simulink model "mrefrobotarm_modified_previous_y_previous_u_previous_ref_Thao"  (R2018b)
settings: Solver=FixedStepAuto  StartTime=0.0  StopTime=10  RelTol=1e-3  AbsTol=1e-6
undefined symbols (not defined in the file or in its folder): sfunxy2
libraries: neural x668, simulink x1
(part 14 of 21)

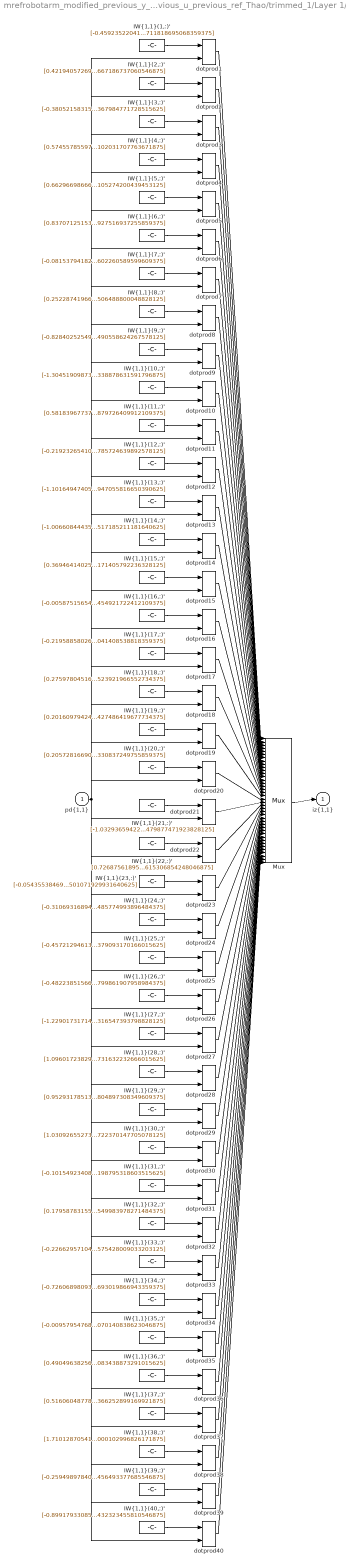
== system mrefrobotarm_modified_previous_y_previous_u_previous_ref_Thao/trimmed_1/Layer 1/IW{1,1} ==
  "pd{1,1}" : Inport  PortDimensions=10
      mask Display: e = 0.06;c1 = [120 230 180]/255;c2 = ([120 230 180]+0)/(256+128);c3 = ([120 230 180]+128)/(256+128);patch([0 1 1 0],[0 0 1 1],c1);patch([0 1 1 1-e 1-e 0+e],[0 0 1 1-e 0+e 0+e],c2);patch([0 0 1 1-e 0+e 0+e],[0 1 1 1-e 1-e 0+e],c3);plot([0 1 1 0 0],[0 0 1 1 0]);
  "IW{1,1}(1,:)'" : Constant  Value=[-0.459235220416795819620148222384159453213214874267578125;-0.29349824568717675088436180885764770209789276123046875;1.04961602685572064075358866830356419086456298828125;0.7919521211983930886191274112206883728504180908203125;-1.1784595378789595176982629709527827799320220947265625;1.1211787526460994524057923626969568431377410888671875;-0.490550798188298220470215937893954105675220489501953125;0.0281424900047358324262081197275620070286095142364501953125;0.443160657725568507547819763203733600676059722900390625;-0.1531042527124218677325728776850155554711818695068359375]
      mask Display: e = 0.06;c1 = [120 150 230]/255;c2 = ([120 150 230]+0)/383;c3 = ([120 150 230]+128)/383;patch([0 1 1 0],[0 0 1 1],c1);patch([0 1 1 1-e 1-e 0+e],[0 0 1 1-e 0+e 0+e],c2);patch([0 0 1 1-e 0+e 0+e],[0 1 1 1-e 1-e 0+e],c3);plot([0 1 1 0 0],[0 0 1 1 0]);disp('Weights');
  "IW{1,1}(10,:)'" : Constant  Value=[-1.304519098736843130126317191752605140209197998046875;-0.306877759776605751884659412098699249327182769775390625;0.5237566266513227208889702524174936115741729736328125;0.10945152834388600926462942197758820839226245880126953125;0.48910555309599768047945644866558723151683807373046875;-1.0719933374810057813419916783459484577178955078125;-0.15974131494668253328228502141428180038928985595703125;0.804989926550838230667750394786708056926727294921875;-0.046877573285782979384261892619178979657590389251708984375;-0.060441319600902036757172908210122841410338878631591796875]
      mask Display: e = 0.06;c1 = [120 150 230]/255;c2 = ([120 150 230]+0)/383;c3 = ([120 150 230]+128)/383;patch([0 1 1 0],[0 0 1 1],c1);patch([0 1 1 1-e 1-e 0+e],[0 0 1 1-e 0+e 0+e],c2);patch([0 0 1 1-e 0+e 0+e],[0 1 1 1-e 1-e 0+e],c3);plot([0 1 1 0 0],[0 0 1 1 0]);disp('Weights');
  "IW{1,1}(11,:)'" : Constant  Value=[0.5818396773725129644816433938103727996349334716796875;-0.0152744671885454534610015997486698324792087078094482421875;-1.3902737988604008112503152005956508219242095947265625;-0.090341627385831457797138455134700052440166473388671875;-0.08192938236897930048829863380888127721846103668212890625;-1.1836377842268201998621179882320575416088104248046875;-0.94837696822625761061686944231041707098484039306640625;0.67302924934781593879762340293382294476032257080078125;0.279503475348413743528652730674366466701030731201171875;-0.7270775313874044964990162043250165879726409912109375]
      mask Display: e = 0.06;c1 = [120 150 230]/255;c2 = ([120 150 230]+0)/383;c3 = ([120 150 230]+128)/383;patch([0 1 1 0],[0 0 1 1],c1);patch([0 1 1 1-e 1-e 0+e],[0 0 1 1-e 0+e 0+e],c2);patch([0 0 1 1-e 0+e 0+e],[0 1 1 1-e 1-e 0+e],c3);plot([0 1 1 0 0],[0 0 1 1 0]);disp('Weights');
  "IW{1,1}(12,:)'" : Constant  Value=[-0.2192326541079176183135501787546672858297824859619140625;0.034961204740979488769792027369476272724568843841552734375;-0.78480877090928391481838843901641666889190673828125;-0.68497188483738924436039496868033893406391143798828125;0.9496056043739018459604039890109561383724212646484375;0.59138070807167919529234723086119629442691802978515625;0.02938148514822198908991168764259782619774341583251953125;0.47042016217384075016383349066018126904964447021484375;0.0528506255461557439279118852937244810163974761962890625;0.8492892171110704158110138450865633785724639892578125]
      mask Display: e = 0.06;c1 = [120 150 230]/255;c2 = ([120 150 230]+0)/383;c3 = ([120 150 230]+128)/383;patch([0 1 1 0],[0 0 1 1],c1);patch([0 1 1 1-e 1-e 0+e],[0 0 1 1-e 0+e 0+e],c2);patch([0 0 1 1-e 0+e 0+e],[0 1 1 1-e 1-e 0+e],c3);plot([0 1 1 0 0],[0 0 1 1 0]);disp('Weights');
  "IW{1,1}(13,:)'" : Constant  Value=[-1.1016494740575859534459368660463951528072357177734375;-0.58886092713398652254142007222981192171573638916015625;-0.7307837342220271370507589381304569542407989501953125;0.7557155236138466403161828566226176917552947998046875;-0.34920491976783851750809617442428134381771087646484375;-0.87052916654144818497940150336944498121738433837890625;-0.1667532157244010215801921503953053615987300872802734375;-0.054286569446526149185228149463000590912997722625732421875;0.241223838878424856613236215707729570567607879638671875;0.700996124572663692475771313183940947055816650390625]
      mask Display: e = 0.06;c1 = [120 150 230]/255;c2 = ([120 150 230]+0)/383;c3 = ([120 150 230]+128)/383;patch([0 1 1 0],[0 0 1 1],c1);patch([0 1 1 1-e 1-e 0+e],[0 0 1 1-e 0+e 0+e],c2);patch([0 0 1 1-e 0+e 0+e],[0 1 1 1-e 1-e 0+e],c3);plot([0 1 1 0 0],[0 0 1 1 0]);disp('Weights');
  "IW{1,1}(14,:)'" : Constant  Value=[-1.006608444357844245331534693832509219646453857421875;-0.35711572844715055996545061134384013712406158447265625;0.32909480035113836127180775292799808084964752197265625;-0.55110276961780180204897305884514935314655303955078125;1.154802213522362563935530488379299640655517578125;0.397605348225490207170196299557574093341827392578125;-0.71574591313160329519860169966705143451690673828125;0.48159191024112935064493967729504220187664031982421875;-0.78679680756141412434345738802221603691577911376953125;-0.441768530810494441940505794264026917517185211181640625]
      mask Display: e = 0.06;c1 = [120 150 230]/255;c2 = ([120 150 230]+0)/383;c3 = ([120 150 230]+128)/383;patch([0 1 1 0],[0 0 1 1],c1);patch([0 1 1 1-e 1-e 0+e],[0 0 1 1-e 0+e 0+e],c2);patch([0 0 1 1-e 0+e 0+e],[0 1 1 1-e 1-e 0+e],c3);plot([0 1 1 0 0],[0 0 1 1 0]);disp('Weights');
  "IW{1,1}(15,:)'" : Constant  Value=[0.369464140250917616459247483362560160458087921142578125;-0.937888588280831658750003043678589165210723876953125;1.0867534228885114000462408512248657643795013427734375;-0.52592004088093335933962180206435732543468475341796875;0.112207093713337424656373286779853515326976776123046875;0.465684224635162069549920715871849097311496734619140625;-0.431210336591754950230637177810422144830226898193359375;-0.303101408244178305295690734055824577808380126953125;-0.69731111958409119910839990552631206810474395751953125;0.08481772702666075247623922450657119043171405792236328125]
      mask Display: e = 0.06;c1 = [120 150 230]/255;c2 = ([120 150 230]+0)/383;c3 = ([120 150 230]+128)/383;patch([0 1 1 0],[0 0 1 1],c1);patch([0 1 1 1-e 1-e 0+e],[0 0 1 1-e 0+e 0+e],c2);patch([0 0 1 1-e 0+e 0+e],[0 1 1 1-e 1-e 0+e],c3);plot([0 1 1 0 0],[0 0 1 1 0]);disp('Weights');
  "IW{1,1}(16,:)'" : Constant  Value=[-0.005875156547677277962815622913694824092090129852294921875;-0.77071460027049354390982216500560753047466278076171875;-1.142444277782478589955417191958986222743988037109375;0.00057501630162004428725719407111682812683284282684326171875;1.1843998886999156372468178233248181641101837158203125;-0.564351201026638715774197407881729304790496826171875;-0.6111872289272748393074152772896923124790191650390625;-0.6547030283798418448526490465155802667140960693359375;-1.1908742302352506303719792413176037371158599853515625;-0.0548431276366504183439332109628594480454921722412109375]
      mask Display: e = 0.06;c1 = [120 150 230]/255;c2 = ([120 150 230]+0)/383;c3 = ([120 150 230]+128)/383;patch([0 1 1 0],[0 0 1 1],c1);patch([0 1 1 1-e 1-e 0+e],[0 0 1 1-e 0+e 0+e],c2);patch([0 0 1 1-e 0+e 0+e],[0 1 1 1-e 1-e 0+e],c3);plot([0 1 1 0 0],[0 0 1 1 0]);disp('Weights');
  "IW{1,1}(17,:)'" : Constant  Value=[-0.2195885802646860562870045896488591097295284271240234375;-0.3575806967372410216654543546610511839389801025390625;0.97143694571848226981813922975561581552028656005859375;-0.8289197498612617120983259155764244496822357177734375;-0.5746253167151700314008166969870217144489288330078125;-0.0506852139293310910428402848992845974862575531005859375;-0.2294990560698609016743176880481769330799579620361328125;0.416849708577010702459375579564948566257953643798828125;-0.87616338373132840455781433774973265826702117919921875;0.08519930707200072672602431111954501830041408538818359375]
      mask Display: e = 0.06;c1 = [120 150 230]/255;c2 = ([120 150 230]+0)/383;c3 = ([120 150 230]+128)/383;patch([0 1 1 0],[0 0 1 1],c1);patch([0 1 1 1-e 1-e 0+e],[0 0 1 1-e 0+e 0+e],c2);patch([0 0 1 1-e 0+e 0+e],[0 1 1 1-e 1-e 0+e],c3);plot([0 1 1 0 0],[0 0 1 1 0]);disp('Weights');
  "IW{1,1}(18,:)'" : Constant  Value=[0.275978045164061158711632515405653975903987884521484375;-0.201844925448067258333395557201583869755268096923828125;0.369878378264276774789465207504690624773502349853515625;0.413333003679872412750029297967557795345783233642578125;0.506360871776887488948659665766172111034393310546875;-0.93265275816585446744255705198156647384166717529296875;-0.0965695424353806008976874863947159610688686370849609375;0.36861066338864378888473538609105162322521209716796875;-0.734700546032511336846937410882674157619476318359375;-0.99055277611612291277509712017490528523921966552734375]
      mask Display: e = 0.06;c1 = [120 150 230]/255;c2 = ([120 150 230]+0)/383;c3 = ([120 150 230]+128)/383;patch([0 1 1 0],[0 0 1 1],c1);patch([0 1 1 1-e 1-e 0+e],[0 0 1 1-e 0+e 0+e],c2);patch([0 0 1 1-e 0+e 0+e],[0 1 1 1-e 1-e 0+e],c3);plot([0 1 1 0 0],[0 0 1 1 0]);disp('Weights');
  "IW{1,1}(19,:)'" : Constant  Value=[0.2016097942440719104073565404178225435316562652587890625;-0.292006737817900929865544412677991203963756561279296875;1.0762677103940505585200071436702273786067962646484375;-0.437529738725115524555775436965632252395153045654296875;1.4057628148362562026107980273081921041011810302734375;-1.0115085483930297272081588744185864925384521484375;1.4608491956607905226661614506156183779239654541015625;-0.0263676635064111104800321783159233746118843555450439453125;-0.560893447360877761553865639143623411655426025390625;0.01126831078487092706319483426113947643898427486419677734375]
      mask Display: e = 0.06;c1 = [120 150 230]/255;c2 = ([120 150 230]+0)/383;c3 = ([120 150 230]+128)/383;patch([0 1 1 0],[0 0 1 1],c1);patch([0 1 1 1-e 1-e 0+e],[0 0 1 1-e 0+e 0+e],c2);patch([0 0 1 1-e 0+e 0+e],[0 1 1 1-e 1-e 0+e],c3);plot([0 1 1 0 0],[0 0 1 1 0]);disp('Weights');
  "IW{1,1}(2,:)'" : Constant  Value=[0.421940572696684224052177114572259597480297088623046875;1.1394047830481301986083053634501993656158447265625;-0.9276428928608384527620955850579775869846343994140625;-0.319621581377210917107589693841873668134212493896484375;0.599161290037102833849758098949678242206573486328125;0.3502538826006265093582214831258170306682586669921875;0.76486814909031386466864432804868556559085845947265625;-0.39442526404542543883025018658372573554515838623046875;0.727514701167386146352100695366971194744110107421875;-0.276969707672654219532404340498032979667186737060546875]
      mask Display: e = 0.06;c1 = [120 150 230]/255;c2 = ([120 150 230]+0)/383;c3 = ([120 150 230]+128)/383;patch([0 1 1 0],[0 0 1 1],c1);patch([0 1 1 1-e 1-e 0+e],[0 0 1 1-e 0+e 0+e],c2);patch([0 0 1 1-e 0+e 0+e],[0 1 1 1-e 1-e 0+e],c3);plot([0 1 1 0 0],[0 0 1 1 0]);disp('Weights');
  "IW{1,1}(20,:)'" : Constant  Value=[0.205728166907649556716108918408281169831752777099609375;0.98978059918219962742824691304122097790241241455078125;0.670105035888260314180797649896703660488128662109375;-0.0727233259149407673671561269657104276120662689208984375;1.153059473829215253459778978140093386173248291015625;0.491497972255601933699864503068965859711170196533203125;-0.69500217773896599826599640437052585184574127197265625;0.85994847944253038907191921680350787937641143798828125;-0.835551186472724527476430012029595673084259033203125;-0.74790216150634802882990470607182942330837249755859375]
      mask Display: e = 0.06;c1 = [120 150 230]/255;c2 = ([120 150 230]+0)/383;c3 = ([120 150 230]+128)/383;patch([0 1 1 0],[0 0 1 1],c1);patch([0 1 1 1-e 1-e 0+e],[0 0 1 1-e 0+e 0+e],c2);patch([0 0 1 1-e 0+e 0+e],[0 1 1 1-e 1-e 0+e],c3);plot([0 1 1 0 0],[0 0 1 1 0]);disp('Weights');
  "IW{1,1}(21,:)'" : Constant  Value=[-1.0329365942279211676435579647659324109554290771484375;0.42458628807360121459879565009032376110553741455078125;0.04618443901148210073426270128038595430552959442138671875;0.9065560967748407250610398477874696254730224609375;0.26648361510755302905550934156053699553012847900390625;0.0884291687942552473433721615947433747351169586181640625;0.61770434825117381816284023443586193025112152099609375;0.4629829983966817774643232041853480041027069091796875;-1.0141119299122414165736927316174842417240142822265625;0.15100917945186254076617160535533912479877471923828125]
      mask Display: e = 0.06;c1 = [120 150 230]/255;c2 = ([120 150 230]+0)/383;c3 = ([120 150 230]+128)/383;patch([0 1 1 0],[0 0 1 1],c1);patch([0 1 1 1-e 1-e 0+e],[0 0 1 1-e 0+e 0+e],c2);patch([0 0 1 1-e 0+e 0+e],[0 1 1 1-e 1-e 0+e],c3);plot([0 1 1 0 0],[0 0 1 1 0]);disp('Weights');
  "IW{1,1}(22,:)'" : Constant  Value=[0.7268756189553073898679258491029031574726104736328125;-0.467689105554118522700690618876251392066478729248046875;1.109281880772417405722762850928120315074920654296875;0.27315022414110179393986754803336225450038909912109375;0.43094504121100218885231925014522857964038848876953125;-0.163097227005093603491303611008333973586559295654296875;0.86284083669027011875840571519802324473857879638671875;0.44549143038833693974964944573002867400646209716796875;0.299238776986608112640197987275314517319202423095703125;-1.12148762799542378587602797779254615306854248046875]
      mask Display: e = 0.06;c1 = [120 150 230]/255;c2 = ([120 150 230]+0)/383;c3 = ([120 150 230]+128)/383;patch([0 1 1 0],[0 0 1 1],c1);patch([0 1 1 1-e 1-e 0+e],[0 0 1 1-e 0+e 0+e],c2);patch([0 0 1 1-e 0+e 0+e],[0 1 1 1-e 1-e 0+e],c3);plot([0 1 1 0 0],[0 0 1 1 0]);disp('Weights');
  "IW{1,1}(23,:)'" : Constant  Value=[-0.0543553846922637806660105752598610706627368927001953125;0.0894024321997811954876311801854171790182590484619140625;-0.73268180455055631483674005721695721149444580078125;-0.87990063776815652385465682527865283191204071044921875;-0.1341766531305843279664458123079384677112102508544921875;0.617144986876134726827558552031405270099639892578125;-0.64440139361752535318572654432500712573528289794921875;-0.5619417681658263052923985014786012470722198486328125;-1.0054577554698818087075551375164650380611419677734375;-0.64369874313411801214357410572119988501071929931640625]
      mask Display: e = 0.06;c1 = [120 150 230]/255;c2 = ([120 150 230]+0)/383;c3 = ([120 150 230]+128)/383;patch([0 1 1 0],[0 0 1 1],c1);patch([0 1 1 1-e 1-e 0+e],[0 0 1 1-e 0+e 0+e],c2);patch([0 0 1 1-e 0+e 0+e],[0 1 1 1-e 1-e 0+e],c3);plot([0 1 1 0 0],[0 0 1 1 0]);disp('Weights');
  "IW{1,1}(24,:)'" : Constant  Value=[-0.31069316894714871235549935590825043618679046630859375;-0.5814084330997444372002291856915690004825592041015625;-0.822688715191450814501195054617710411548614501953125;-0.1990172295149660597335383727113367058336734771728515625;-0.253642741079357747491229702063719742000102996826171875;1.2263993908007790878400555811822414398193359375;-1.0833193209512239629788155070855282247066497802734375;-0.7328344121728693760786654820549301803112030029296875;-0.466145811881534422038697584866895340383052825927734375;0.67576516762366212187629344043671153485774993896484375]
      mask Display: e = 0.06;c1 = [120 150 230]/255;c2 = ([120 150 230]+0)/383;c3 = ([120 150 230]+128)/383;patch([0 1 1 0],[0 0 1 1],c1);patch([0 1 1 1-e 1-e 0+e],[0 0 1 1-e 0+e 0+e],c2);patch([0 0 1 1-e 0+e 0+e],[0 1 1 1-e 1-e 0+e],c3);plot([0 1 1 0 0],[0 0 1 1 0]);disp('Weights');
  "IW{1,1}(25,:)'" : Constant  Value=[-0.457212946136130060637015048996545374393463134765625;-0.7632016106977881353401471642428077757358551025390625;0.248761073438853286265981523683876730501651763916015625;-0.82845030997187818488924904158920980989933013916015625;0.505824858023265822026814930723048746585845947265625;-0.07525956372700999541525135327901807613670825958251953125;-0.43507647282099137786559595042490400373935699462890625;0.1433382425757481204442456146352924406528472900390625;-1.012707980842789456943364712060429155826568603515625;1.0154921878932070544721000260324217379093170166015625]
      mask Display: e = 0.06;c1 = [120 150 230]/255;c2 = ([120 150 230]+0)/383;c3 = ([120 150 230]+128)/383;patch([0 1 1 0],[0 0 1 1],c1);patch([0 1 1 1-e 1-e 0+e],[0 0 1 1-e 0+e 0+e],c2);patch([0 0 1 1-e 0+e 0+e],[0 1 1 1-e 1-e 0+e],c3);plot([0 1 1 0 0],[0 0 1 1 0]);disp('Weights');
  "IW{1,1}(26,:)'" : Constant  Value=[-0.482238515660687594444056003339937888085842132568359375;0.43664743448262222091926787470583803951740264892578125;0.9059650556878284799466882759588770568370819091796875;0.99126888040064786711269562147208489477634429931640625;0.68645376393967760808578759679221548140048980712890625;0.436805971255550928855626580116222612559795379638671875;0.52149439943570008448858743577147834002971649169921875;-1.147843483439997758210893152863718569278717041015625;-0.6869851111536575682947614041040651500225067138671875;-0.4622743181047521687787593691609799861907958984375]
      mask Display: e = 0.06;c1 = [120 150 230]/255;c2 = ([120 150 230]+0)/383;c3 = ([120 150 230]+128)/383;patch([0 1 1 0],[0 0 1 1],c1);patch([0 1 1 1-e 1-e 0+e],[0 0 1 1-e 0+e 0+e],c2);patch([0 0 1 1-e 0+e 0+e],[0 1 1 1-e 1-e 0+e],c3);plot([0 1 1 0 0],[0 0 1 1 0]);disp('Weights');
  "IW{1,1}(27,:)'" : Constant  Value=[-1.2290173171406657548487828535144217312335968017578125;-0.339693794909226742806396259766188450157642364501953125;-1.3099872102940011142635512442211620509624481201171875;0.482428640178804324367689559949212707579135894775390625;-0.787426429106807379554311410174705088138580322265625;-1.290630226961940518748406248050741851329803466796875;-0.636294904372121106206350305001251399517059326171875;-0.8429746733754657217474459685035981237888336181640625;0.84112748843849838298325494179152883589267730712890625;-0.85706488054134855048005192657001316547393798828125]
      mask Display: e = 0.06;c1 = [120 150 230]/255;c2 = ([120 150 230]+0)/383;c3 = ([120 150 230]+128)/383;patch([0 1 1 0],[0 0 1 1],c1);patch([0 1 1 1-e 1-e 0+e],[0 0 1 1-e 0+e 0+e],c2);patch([0 0 1 1-e 0+e 0+e],[0 1 1 1-e 1-e 0+e],c3);plot([0 1 1 0 0],[0 0 1 1 0]);disp('Weights');
  "IW{1,1}(28,:)'" : Constant  Value=[1.0960172382970032600724152871407568454742431640625;1.11928020809361239429335910244844853878021240234375;1.202386667710628298522124168812297284603118896484375;1.0481612806558129324940864535165019333362579345703125;-0.62862547936817936289344288525171577930450439453125;0.93311071875859197266578348717303015291690826416015625;-0.11056156337211316131874383472677436657249927520751953125;-0.2180510108376263189722266133685479871928691864013671875;0.148398225291466678843477211557910777628421783447265625;0.283492187955392493936557229972095228731632232666015625]
      mask Display: e = 0.06;c1 = [120 150 230]/255;c2 = ([120 150 230]+0)/383;c3 = ([120 150 230]+128)/383;patch([0 1 1 0],[0 0 1 1],c1);patch([0 1 1 1-e 1-e 0+e],[0 0 1 1-e 0+e 0+e],c2);patch([0 0 1 1-e 0+e 0+e],[0 1 1 1-e 1-e 0+e],c3);plot([0 1 1 0 0],[0 0 1 1 0]);disp('Weights');
  "IW{1,1}(29,:)'" : Constant  Value=[0.95293178513860443690219881318625994026660919189453125;0.33133892095905637109609642720897682011127471923828125;0.483338481554557886088474560892791487276554107666015625;-0.51936482222186708401778787447256036102771759033203125;-0.26972622615172070492661759999464266002178192138671875;0.32030555728812049043341403375961817800998687744140625;0.8476970920629707251237050513736903667449951171875;0.55373661950981034607366382260806858539581298828125;0.48124014203928699995316264903522096574306488037109375;-1.0822549680681614603372509009204804897308349609375]
      mask Display: e = 0.06;c1 = [120 150 230]/255;c2 = ([120 150 230]+0)/383;c3 = ([120 150 230]+128)/383;patch([0 1 1 0],[0 0 1 1],c1);patch([0 1 1 1-e 1-e 0+e],[0 0 1 1-e 0+e 0+e],c2);patch([0 0 1 1-e 0+e 0+e],[0 1 1 1-e 1-e 0+e],c3);plot([0 1 1 0 0],[0 0 1 1 0]);disp('Weights');
  "IW{1,1}(3,:)'" : Constant  Value=[-0.380521583150016440288965213767369277775287628173828125;-0.1953317707677943160238243081039399839937686920166015625;-1.15548358889821134454223283682949841022491455078125;-0.62498377206752830925751140966895036399364471435546875;0.0507087797953804653161569149233400821685791015625;-0.34993783786551591052926823977031745016574859619140625;-0.3244212476909444919925817885086871683597564697265625;-0.708210613127198573835130446241237223148345947265625;-1.001507019035198897682903407257981598377227783203125;-0.74713690461068138493061496774316765367984771728515625]
      mask Display: e = 0.06;c1 = [120 150 230]/255;c2 = ([120 150 230]+0)/383;c3 = ([120 150 230]+128)/383;patch([0 1 1 0],[0 0 1 1],c1);patch([0 1 1 1-e 1-e 0+e],[0 0 1 1-e 0+e 0+e],c2);patch([0 0 1 1-e 0+e 0+e],[0 1 1 1-e 1-e 0+e],c3);plot([0 1 1 0 0],[0 0 1 1 0]);disp('Weights');
  "IW{1,1}(30,:)'" : Constant  Value=[1.0309265527383129068539346917532384395599365234375;0.0413606629452887009090744641071069054305553436279296875;-0.3228830517519514220481369193294085562229156494140625;0.29760260984668185368917647792841307818889617919921875;-1.946545515298652606617224591900594532489776611328125;0.3727935893046432358488573299837298691272735595703125;0.80546420261760742764778342461795546114444732666015625;-0.10782265636587108625921160864891135133802890777587890625;-0.319428546159855664132720676207100041210651397705078125;-0.059266322181003083802153241776977665722370147705078125]
      mask Display: e = 0.06;c1 = [120 150 230]/255;c2 = ([120 150 230]+0)/383;c3 = ([120 150 230]+128)/383;patch([0 1 1 0],[0 0 1 1],c1);patch([0 1 1 1-e 1-e 0+e],[0 0 1 1-e 0+e 0+e],c2);patch([0 0 1 1-e 0+e 0+e],[0 1 1 1-e 1-e 0+e],c3);plot([0 1 1 0 0],[0 0 1 1 0]);disp('Weights');
  "IW{1,1}(31,:)'" : Constant  Value=[-0.10154923408813874841083446654010913334786891937255859375;0.10463337133623425156958575144017231650650501251220703125;-0.70847745109132576057930918977945111691951751708984375;0.027565213845020038185840149935756926424801349639892578125;1.30488787423937591114508904865942895412445068359375;-0.4519431314107926755951893937890417873859405517578125;-0.6772719404750320304486876921146176755428314208984375;0.54505973361519977071765197251806966960430145263671875;-0.51117067626427237225783528629108332097530364990234375;-1.210078878158766801931278678239323198795318603515625]
      mask Display: e = 0.06;c1 = [120 150 230]/255;c2 = ([120 150 230]+0)/383;c3 = ([120 150 230]+128)/383;patch([0 1 1 0],[0 0 1 1],c1);patch([0 1 1 1-e 1-e 0+e],[0 0 1 1-e 0+e 0+e],c2);patch([0 0 1 1-e 0+e 0+e],[0 1 1 1-e 1-e 0+e],c3);plot([0 1 1 0 0],[0 0 1 1 0]);disp('Weights');
  "IW{1,1}(32,:)'" : Constant  Value=[0.179587831554380017440308847653795965015888214111328125;0.7883086760053081842869460160727612674236297607421875;0.0849530317101877263663567418916500173509120941162109375;-0.97114080450967932289785267130355350673198699951171875;-0.68829519715637232923910460158367641270160675048828125;0.1382223600981604405557590098396758548915386199951171875;0.0650971082997748029530526991948136128485202789306640625;-0.97912539307000157062788048278889618813991546630859375;0.377737036819926930153457078631618060171604156494140625;-0.037257089605611769245196995825608610175549983978271484375]
      mask Display: e = 0.06;c1 = [120 150 230]/255;c2 = ([120 150 230]+0)/383;c3 = ([120 150 230]+128)/383;patch([0 1 1 0],[0 0 1 1],c1);patch([0 1 1 1-e 1-e 0+e],[0 0 1 1-e 0+e 0+e],c2);patch([0 0 1 1-e 0+e 0+e],[0 1 1 1-e 1-e 0+e],c3);plot([0 1 1 0 0],[0 0 1 1 0]);disp('Weights');
  "IW{1,1}(33,:)'" : Constant  Value=[-0.22662957104480419001646396282012574374675750732421875;0.72844507586478102201255069303442724049091339111328125;0.6141592781255564847953110074740834534168243408203125;0.101220068298868592915340514082345180213451385498046875;-1.30038356567382695772039369330741465091705322265625;0.1760612213506755063807673877818160690367221832275390625;-0.6234508806817145032397320392192341387271881103515625;0.2578514765769128747052718608756549656391143798828125;-0.498938688455254297782204275790718384087085723876953125;-0.60798051305062739135820493174833245575428009033203125]
      mask Display: e = 0.06;c1 = [120 150 230]/255;c2 = ([120 150 230]+0)/383;c3 = ([120 150 230]+128)/383;patch([0 1 1 0],[0 0 1 1],c1);patch([0 1 1 1-e 1-e 0+e],[0 0 1 1-e 0+e 0+e],c2);patch([0 0 1 1-e 0+e 0+e],[0 1 1 1-e 1-e 0+e],c3);plot([0 1 1 0 0],[0 0 1 1 0]);disp('Weights');
  "IW{1,1}(34,:)'" : Constant  Value=[-0.72606898093604288479951947010704316198825836181640625;-0.2483973014773266374533022826653905212879180908203125;0.3447701180893443240194073950988240540027618408203125;-0.535603816887748163111382382339797914028167724609375;-1.3458614133875206331225626854575239121913909912109375;-0.8760247396851033041542677892721258103847503662109375;0.051268955020888802576184417603144538588821887969970703125;-0.100179505101124333155127033023745752871036529541015625;0.77567804361125503032070582776213996112346649169921875;-1.067527970594736697051985174766741693019866943359375]
      mask Display: e = 0.06;c1 = [120 150 230]/255;c2 = ([120 150 230]+0)/383;c3 = ([120 150 230]+128)/383;patch([0 1 1 0],[0 0 1 1],c1);patch([0 1 1 1-e 1-e 0+e],[0 0 1 1-e 0+e 0+e],c2);patch([0 0 1 1-e 0+e 0+e],[0 1 1 1-e 1-e 0+e],c3);plot([0 1 1 0 0],[0 0 1 1 0]);disp('Weights');
  "IW{1,1}(35,:)'" : Constant  Value=[-0.009579547688245003411733335951794288121163845062255859375;-0.29752550499882712831123399155330844223499298095703125;0.65143322006700332682527232464053668081760406494140625;0.332652536277042887302712870223331265151500701904296875;-2.2272030138975953406088592601008713245391845703125;1.0653879429574981685391321661882102489471435546875;0.21910403774254760822515208928962238132953643798828125;0.56979557384155044008622326145996339619159698486328125;-0.457860103534204088138181987233110703527927398681640625;0.09151087536235451291855014233078691177070140838623046875]
      mask Display: e = 0.06;c1 = [120 150 230]/255;c2 = ([120 150 230]+0)/383;c3 = ([120 150 230]+128)/383;patch([0 1 1 0],[0 0 1 1],c1);patch([0 1 1 1-e 1-e 0+e],[0 0 1 1-e 0+e 0+e],c2);patch([0 0 1 1-e 0+e 0+e],[0 1 1 1-e 1-e 0+e],c3);plot([0 1 1 0 0],[0 0 1 1 0]);disp('Weights');
  "IW{1,1}(36,:)'" : Constant  Value=[0.490496382567982946998341731159598566591739654541015625;0.5140979931972555760921750334091484546661376953125;-0.8988053057708096371669626023503951728343963623046875;0.6604036565352171539444725567591376602649688720703125;0.15330915046754978181553497051936574280261993408203125;-0.1642381880988101061635831001694896258413791656494140625;-0.8062262031936218154015705295023508369922637939453125;-0.5572652561952178285054060324910096824169158935546875;0.0231050938200449140769165978781529702246189117431640625;-0.4410080082838929715904896511347033083438873291015625]
      mask Display: e = 0.06;c1 = [120 150 230]/255;c2 = ([120 150 230]+0)/383;c3 = ([120 150 230]+128)/383;patch([0 1 1 0],[0 0 1 1],c1);patch([0 1 1 1-e 1-e 0+e],[0 0 1 1-e 0+e 0+e],c2);patch([0 0 1 1-e 0+e 0+e],[0 1 1 1-e 1-e 0+e],c3);plot([0 1 1 0 0],[0 0 1 1 0]);disp('Weights');
  "IW{1,1}(37,:)'" : Constant  Value=[0.516060487788239097284304079948924481868743896484375;-0.94460255007425786288877134211361408233642578125;-0.95344586556598664994766068048193119466304779052734375;0.480311068714104283383647953087347559630870819091796875;0.9186881888995699352307156004826538264751434326171875;0.58003412464287495975412412008154205977916717529296875;0.0219738035054113690913712986230166279710829257965087890625;-0.72419254803511334817045508316368795931339263916015625;-0.52677042105196936194744239401188679039478302001953125;-0.439266919696432445174849590330268256366252899169921875]
      mask Display: e = 0.06;c1 = [120 150 230]/255;c2 = ([120 150 230]+0)/383;c3 = ([120 150 230]+128)/383;patch([0 1 1 0],[0 0 1 1],c1);patch([0 1 1 1-e 1-e 0+e],[0 0 1 1-e 0+e 0+e],c2);patch([0 0 1 1-e 0+e 0+e],[0 1 1 1-e 1-e 0+e],c3);plot([0 1 1 0 0],[0 0 1 1 0]);disp('Weights');
  "IW{1,1}(38,:)'" : Constant  Value=[1.7101287054125517972380521314335055649280548095703125;1.7737639049575724126128761781728826463222503662109375;0.85894090225937713700687936579925008118152618408203125;0.381842805121030526294134688214398920536041259765625;1.566925055542294220600751941674388945102691650390625;0.63434261904892241812348174789804033935070037841796875;1.17979714902582966118416152312420308589935302734375;0.97507425789570778551507146403309889137744903564453125;-0.003862134050635519788574612221054849214851856231689453125;-1.198213154482018705238033362547867000102996826171875]
      mask Display: e = 0.06;c1 = [120 150 230]/255;c2 = ([120 150 230]+0)/383;c3 = ([120 150 230]+128)/383;patch([0 1 1 0],[0 0 1 1],c1);patch([0 1 1 1-e 1-e 0+e],[0 0 1 1-e 0+e 0+e],c2);patch([0 0 1 1-e 0+e 0+e],[0 1 1 1-e 1-e 0+e],c3);plot([0 1 1 0 0],[0 0 1 1 0]);disp('Weights');
  "IW{1,1}(39,:)'" : Constant  Value=[-0.2594989784082983863555682546575553715229034423828125;-0.09506918862064084319030143888085149228572845458984375;0.165650774548008694608824953320436179637908935546875;-0.7095939350563522651782477623783051967620849609375;-1.095557923289508295283667393960058689117431640625;-0.2349190676622031348497188218971132300794124603271484375;-0.205176988321424558225913870046497322618961334228515625;0.73900360397848141591481407886021770536899566650390625;0.441395758661922987808878815485513769090175628662109375;0.760614206598187347907469302299432456493377685546875]
      mask Display: e = 0.06;c1 = [120 150 230]/255;c2 = ([120 150 230]+0)/383;c3 = ([120 150 230]+128)/383;patch([0 1 1 0],[0 0 1 1],c1);patch([0 1 1 1-e 1-e 0+e],[0 0 1 1-e 0+e 0+e],c2);patch([0 0 1 1-e 0+e 0+e],[0 1 1 1-e 1-e 0+e],c3);plot([0 1 1 0 0],[0 0 1 1 0]);disp('Weights');
  "IW{1,1}(4,:)'" : Constant  Value=[0.5745578559796948869831112460815347731113433837890625;0.43594646779250922907777976433862932026386260986328125;0.78145780110102325277665613612043671309947967529296875;0.7809240139169180139333548140712082386016845703125;-0.757931918994925180044219814590178430080413818359375;0.42532150546884828212768070443416945636272430419921875;0.5658538182308323616354073237744159996509552001953125;-0.52860671081283128192040976500720717012882232666015625;-0.28198389483756181039808552668546326458454132080078125;0.68198059347156003706658111696015112102031707763671875]
      mask Display: e = 0.06;c1 = [120 150 230]/255;c2 = ([120 150 230]+0)/383;c3 = ([120 150 230]+128)/383;patch([0 1 1 0],[0 0 1 1],c1);patch([0 1 1 1-e 1-e 0+e],[0 0 1 1-e 0+e 0+e],c2);patch([0 0 1 1-e 0+e 0+e],[0 1 1 1-e 1-e 0+e],c3);plot([0 1 1 0 0],[0 0 1 1 0]);disp('Weights');
  "IW{1,1}(40,:)'" : Constant  Value=[-0.89917933085833168238565349383861757814884185791015625;-0.655418209159318365664148586802184581756591796875;0.79131564665822284876384173912811093032360076904296875;-0.32995307800854067892259990912862122058868408203125;-0.599878580415268647385573785868473351001739501953125;0.540655473554314536244191913283430039882659912109375;-0.2179751347957027685087183499490492977201938629150390625;1.0751657453224847671435782103799283504486083984375;-0.262585064145549218483921549704973585903644561767578125;-0.92522154860780669860531588710728101432323455810546875]
      mask Display: e = 0.06;c1 = [120 150 230]/255;c2 = ([120 150 230]+0)/383;c3 = ([120 150 230]+128)/383;patch([0 1 1 0],[0 0 1 1],c1);patch([0 1 1 1-e 1-e 0+e],[0 0 1 1-e 0+e 0+e],c2);patch([0 0 1 1-e 0+e 0+e],[0 1 1 1-e 1-e 0+e],c3);plot([0 1 1 0 0],[0 0 1 1 0]);disp('Weights');
  "IW{1,1}(5,:)'" : Constant  Value=[0.662966986667456570359036049921996891498565673828125;0.28682195138465471639932502512237988412380218505859375;1.1762255773689478388632778660394251346588134765625;0.9945704745068619789805097752832807600498199462890625;-0.85014879069712090409183247174951247870922088623046875;0.1649293009150895328307484533070237375795841217041015625;0.61936827707909813955922118111629970371723175048828125;0.50663309917842103136109699335065670311450958251953125;-0.6873442064592520939214637110126204788684844970703125;0.427177855605174461306461353160557337105274200439453125]
      mask Display: e = 0.06;c1 = [120 150 230]/255;c2 = ([120 150 230]+0)/383;c3 = ([120 150 230]+128)/383;patch([0 1 1 0],[0 0 1 1],c1);patch([0 1 1 1-e 1-e 0+e],[0 0 1 1-e 0+e 0+e],c2);patch([0 0 1 1-e 0+e 0+e],[0 1 1 1-e 1-e 0+e],c3);plot([0 1 1 0 0],[0 0 1 1 0]);disp('Weights');
  "IW{1,1}(6,:)'" : Constant  Value=[0.83707125153155903518609193270094692707061767578125;-0.345955447797594850545266353947226889431476593017578125;-0.9503936970261646077773320939741097390651702880859375;0.505832192010364334322503054863773286342620849609375;-0.57086571764714888477243448505760170519351959228515625;0.67050148856771130123632929098675958812236785888671875;0.53862341985638284569404277135618031024932861328125;-0.89073095329790585861218232821556739509105682373046875;0.77848722142508186561116190205211751163005828857421875;0.2070769098838173005727725239921710453927516937255859375]
      mask Display: e = 0.06;c1 = [120 150 230]/255;c2 = ([120 150 230]+0)/383;c3 = ([120 150 230]+128)/383;patch([0 1 1 0],[0 0 1 1],c1);patch([0 1 1 1-e 1-e 0+e],[0 0 1 1-e 0+e 0+e],c2);patch([0 0 1 1-e 0+e 0+e],[0 1 1 1-e 1-e 0+e],c3);plot([0 1 1 0 0],[0 0 1 1 0]);disp('Weights');
  "IW{1,1}(7,:)'" : Constant  Value=[-0.0815379418245985865265623715458787046372890472412109375;-0.6582587897791432052230220506316982209682464599609375;0.31871821424702428959818689691019244492053985595703125;0.36699039613368966694650907811592333018779754638671875;0.3556971133670738804966049428912810981273651123046875;1.08859421033406977841195839573629200458526611328125;0.5929898168935350266650630146614275872707366943359375;-0.394796973334014034140437843234394676983356475830078125;0.46014365857287120586960327273118309676647186279296875;0.03128507764742226304743866194257861934602260589599609375]
      mask Display: e = 0.06;c1 = [120 150 230]/255;c2 = ([120 150 230]+0)/383;c3 = ([120 150 230]+128)/383;patch([0 1 1 0],[0 0 1 1],c1);patch([0 1 1 1-e 1-e 0+e],[0 0 1 1-e 0+e 0+e],c2);patch([0 0 1 1-e 0+e 0+e],[0 1 1 1-e 1-e 0+e],c3);plot([0 1 1 0 0],[0 0 1 1 0]);disp('Weights');
  "IW{1,1}(8,:)'" : Constant  Value=[0.252287419667901080533312097031739540398120880126953125;0.39448386787555367316571164337801747024059295654296875;-0.7778828916612774424521603577886708080768585205078125;0.67369428825519361847540267262957058846950531005859375;0.0272763648776374843796244107352322316728532314300537109375;-0.94929720088395985744256222460535354912281036376953125;0.94218604191232468991756832110695540904998779296875;-0.433281811325026688930250884368433617055416107177734375;1.0797015724823200155668700972455553710460662841796875;-0.06162190747630176546056901543124695308506488800048828125]
      mask Display: e = 0.06;c1 = [120 150 230]/255;c2 = ([120 150 230]+0)/383;c3 = ([120 150 230]+128)/383;patch([0 1 1 0],[0 0 1 1],c1);patch([0 1 1 1-e 1-e 0+e],[0 0 1 1-e 0+e 0+e],c2);patch([0 0 1 1-e 0+e 0+e],[0 1 1 1-e 1-e 0+e],c3);plot([0 1 1 0 0],[0 0 1 1 0]);disp('Weights');
  "IW{1,1}(9,:)'" : Constant  Value=[-0.828402525497675679133635640027932822704315185546875;0.6657276651966250735625862944289110600948333740234375;-0.165790510194598172954982828741776756942272186279296875;0.040376384442278610842347319476175471208989620208740234375;-0.73235285901514812767487683231593109667301177978515625;-0.547913141658167734959761219215579330921173095703125;-0.7885715628427760748309083282947540283203125;-0.8010959759390250400912236727890558540821075439453125;-0.413564682216540913106683774458360858261585235595703125;0.85293091872862369928753878411953337490558624267578125]
      mask Display: e = 0.06;c1 = [120 150 230]/255;c2 = ([120 150 230]+0)/383;c3 = ([120 150 230]+128)/383;patch([0 1 1 0],[0 0 1 1],c1);patch([0 1 1 1-e 1-e 0+e],[0 0 1 1-e 0+e 0+e],c2);patch([0 0 1 1-e 0+e 0+e],[0 1 1 1-e 1-e 0+e],c3);plot([0 1 1 0 0],[0 0 1 1 0]);disp('Weights');
  Mux : Mux  Inputs=40
      mask Display: e = 0.06;c1 = [120 150 230]/255;c2 = ([120 150 230]+0)/383;c3 = ([120 150 230]+128)/383;patch([0 1 1 0],[0 0 1 1],c1);patch([0 1 1 1-e 1-e 0+e],[0 0 1 1-e 0+e 0+e],c2);patch([0 0 1 1-e 0+e 0+e],[0 1 1 1-e 1-e 0+e],c3);plot([0 1 1 0 0],[0 0 1 1 0]);disp('Mux');
  dotprod{1..40} (40 alike) : neural/Weight Functions/dotprod
  "iz{1,1}" : Outport
      mask Display: e = 0.06;c1 = [120 230 180]/255;c2 = ([120 230 180]+0)/(256+128);c3 = ([120 230 180]+128)/(256+128);patch([0 1 1 0],[0 0 1 1],c1);patch([0 1 1 1-e 1-e 0+e],[0 0 1 1-e 0+e 0+e],c2);patch([0 0 1 1-e 0+e 0+e],[0 1 1 1-e 1-e 0+e],c3);plot([0 1 1 0 0],[0 0 1 1 0]);
  wires:
  "IW{1,1}(1,:)'"/1 -> dotprod1/1
  "pd{1,1}"/1 -> dotprod1/2, dotprod2/2, dotprod3/2, dotprod4/2, dotprod5/2, dotprod6/2, dotprod7/2, dotprod8/2, dotprod9/2, dotprod10/2, dotprod11/2, dotprod12/2, dotprod13/2, dotprod14/2, dotprod15/2, dotprod16/2, dotprod17/2, dotprod18/2, dotprod19/2, dotprod20/2, dotprod21/2, dotprod22/2, dotprod23/2, dotprod24/2, dotprod25/2, dotprod26/2, dotprod27/2, dotprod28/2, dotprod29/2, dotprod30/2, dotprod31/2, dotprod32/2, dotprod33/2, dotprod34/2, dotprod35/2, dotprod36/2, dotprod37/2, dotprod38/2, dotprod39/2, dotprod40/2
  dotprod1/1 -> Mux/1
  "IW{1,1}(2,:)'"/1 -> dotprod2/1
  dotprod2/1 -> Mux/2
  "IW{1,1}(3,:)'"/1 -> dotprod3/1
  dotprod3/1 -> Mux/3
  "IW{1,1}(4,:)'"/1 -> dotprod4/1
  dotprod4/1 -> Mux/4
  "IW{1,1}(5,:)'"/1 -> dotprod5/1
  dotprod5/1 -> Mux/5
  "IW{1,1}(6,:)'"/1 -> dotprod6/1
  dotprod6/1 -> Mux/6
  "IW{1,1}(7,:)'"/1 -> dotprod7/1
  dotprod7/1 -> Mux/7
  "IW{1,1}(8,:)'"/1 -> dotprod8/1
  dotprod8/1 -> Mux/8
  "IW{1,1}(9,:)'"/1 -> dotprod9/1
  dotprod9/1 -> Mux/9
  "IW{1,1}(10,:)'"/1 -> dotprod10/1
  dotprod10/1 -> Mux/10
  "IW{1,1}(11,:)'"/1 -> dotprod11/1
  dotprod11/1 -> Mux/11
  "IW{1,1}(12,:)'"/1 -> dotprod12/1
  dotprod12/1 -> Mux/12
  "IW{1,1}(13,:)'"/1 -> dotprod13/1
  dotprod13/1 -> Mux/13
  "IW{1,1}(14,:)'"/1 -> dotprod14/1
  dotprod14/1 -> Mux/14
  "IW{1,1}(15,:)'"/1 -> dotprod15/1
  dotprod15/1 -> Mux/15
  "IW{1,1}(16,:)'"/1 -> dotprod16/1
  dotprod16/1 -> Mux/16
  "IW{1,1}(17,:)'"/1 -> dotprod17/1
  dotprod17/1 -> Mux/17
  "IW{1,1}(18,:)'"/1 -> dotprod18/1
  dotprod18/1 -> Mux/18
  "IW{1,1}(19,:)'"/1 -> dotprod19/1
  dotprod19/1 -> Mux/19
  "IW{1,1}(20,:)'"/1 -> dotprod20/1
  dotprod20/1 -> Mux/20
  "IW{1,1}(21,:)'"/1 -> dotprod21/1
  dotprod21/1 -> Mux/21
  "IW{1,1}(22,:)'"/1 -> dotprod22/1
  dotprod22/1 -> Mux/22
  "IW{1,1}(23,:)'"/1 -> dotprod23/1
  dotprod23/1 -> Mux/23
  "IW{1,1}(24,:)'"/1 -> dotprod24/1
  dotprod24/1 -> Mux/24
  "IW{1,1}(25,:)'"/1 -> dotprod25/1
  dotprod25/1 -> Mux/25
  "IW{1,1}(26,:)'"/1 -> dotprod26/1
  dotprod26/1 -> Mux/26
  "IW{1,1}(27,:)'"/1 -> dotprod27/1
  dotprod27/1 -> Mux/27
  "IW{1,1}(28,:)'"/1 -> dotprod28/1
  dotprod28/1 -> Mux/28
  "IW{1,1}(29,:)'"/1 -> dotprod29/1
  dotprod29/1 -> Mux/29
  "IW{1,1}(30,:)'"/1 -> dotprod30/1
  dotprod30/1 -> Mux/30
  "IW{1,1}(31,:)'"/1 -> dotprod31/1
  dotprod31/1 -> Mux/31
  "IW{1,1}(32,:)'"/1 -> dotprod32/1
  dotprod32/1 -> Mux/32
  "IW{1,1}(33,:)'"/1 -> dotprod33/1
  dotprod33/1 -> Mux/33
  "IW{1,1}(34,:)'"/1 -> dotprod34/1
  dotprod34/1 -> Mux/34
  "IW{1,1}(35,:)'"/1 -> dotprod35/1
  dotprod35/1 -> Mux/35
  "IW{1,1}(36,:)'"/1 -> dotprod36/1
  dotprod36/1 -> Mux/36
  "IW{1,1}(37,:)'"/1 -> dotprod37/1
  dotprod37/1 -> Mux/37
  "IW{1,1}(38,:)'"/1 -> dotprod38/1
  dotprod38/1 -> Mux/38
  "IW{1,1}(39,:)'"/1 -> dotprod39/1
  dotprod39/1 -> Mux/39
  "IW{1,1}(40,:)'"/1 -> dotprod40/1
  dotprod40/1 -> Mux/40
  Mux/1 -> "iz{1,1}"/1

== system mrefrobotarm_modified_previous_y_previous_u_previous_ref_Thao/trimmed_1/Layer 2/Delays 1 ==
  "p{2}" : Inport  PortDimensions=40
      mask Display: e = 0.06;c1 = [120 230 180]/255;c2 = ([120 230 180]+0)/(256+128);c3 = ([120 230 180]+128)/(256+128);patch([0 1 1 0],[0 0 1 1],c1);patch([0 1 1 1-e 1-e 0+e],[0 0 1 1-e 0+e 0+e],c2);patch([0 0 1 1-e 0+e 0+e],[0 1 1 1-e 1-e 0+e],c3);plot([0 1 1 0 0],[0 0 1 1 0]);
  mux : Mux  Inputs=1
      mask Display: e = 0.06;c1 = [120 150 230]/255;c2 = ([120 150 230]+0)/383;c3 = ([120 150 230]+128)/383;patch([0 1 1 0],[0 0 1 1],c1);patch([0 1 1 1-e 1-e 0+e],[0 0 1 1-e 0+e 0+e],c2);patch([0 0 1 1-e 0+e 0+e],[0 1 1 1-e 1-e 0+e],c3);plot([0 1 1 0 0],[0 0 1 1 0]);disp('Mux')
  "pd{2,1}" : Outport
      mask Display: e = 0.06;c1 = [120 230 180]/255;c2 = ([120 230 180]+0)/(256+128);c3 = ([120 230 180]+128)/(256+128);patch([0 1 1 0],[0 0 1 1],c1);patch([0 1 1 1-e 1-e 0+e],[0 0 1 1-e 0+e 0+e],c2);patch([0 0 1 1-e 0+e 0+e],[0 1 1 1-e 1-e 0+e],c3);plot([0 1 1 0 0],[0 0 1 1 0]);
  wires:
  "p{2}"/1 -> mux/1
  mux/1 -> "pd{2,1}"/1

== system mrefrobotarm_modified_previous_y_previous_u_previous_ref_Thao/trimmed_1/Layer 2/LW{2,1} ==
  "ad{2,1}" : Inport  PortDimensions=40
      mask Display: e = 0.06;c1 = [120 230 180]/255;c2 = ([120 230 180]+0)/(256+128);c3 = ([120 230 180]+128)/(256+128);patch([0 1 1 0],[0 0 1 1],c1);patch([0 1 1 1-e 1-e 0+e],[0 0 1 1-e 0+e 0+e],c2);patch([0 0 1 1-e 0+e 0+e],[0 1 1 1-e 1-e 0+e],c3);plot([0 1 1 0 0],[0 0 1 1 0]);
  "IW{2,1}(1,:)'" : Constant  Value=[0.376988242742819223973782527536968700587749481201171875;-0.048983758772740505771370322918301098980009555816650390625;0.053990013334553881019228782633945229463279247283935546875;-0.09726086132984257393019333903794176876544952392578125;0.002474580889355315616029429293121211230754852294921875;0.541869017345185444156641096924431622028350830078125;-0.378939362281856595426887679423089139163494110107421875;-0.83355565275971954530831453666905872523784637451171875;-0.00093369429163297807013066620385188798536546528339385986328125;0.005693258062771836859605745218004813068546354770660400390625;-0.271110000696748010273751106069539673626422882080078125;0.94715123228040531966342996383900754153728485107421875;-0.06761118440421280684216043255219119600951671600341796875;-0.65179245010877917554381610898417420685291290283203125;0.1624081169309350702878447236798820085823535919189453125;-0.74401684175596993764401076987269334495067596435546875;0.1814946143806416556376603921307832933962345123291015625;0.8470651394712305215506376043776981532573699951171875;-0.5302435911462832773821673981728963553905487060546875;-0.0876348579999971233345235077649704180657863616943359375;-0.2029541139761243118133648977163829840719699859619140625;0.258266297126318156163193862084881402552127838134765625;-0.0175908033538817176744117887210450135171413421630859375;0.78715742488328144244036366217187605798244476318359375;0.05362184817972105721484155083089717663824558258056640625;-0.0824899455079083632202952003353857435286045074462890625;-0.01018400514173275518692296515155248926021158695220947265625;0.022859789691910430142751664561728830449283123016357421875;0.029421651302660466187344212585230707190930843353271484375;0.8797171343227068174286387147731147706508636474609375;-0.206428483736689816208098591232555918395519256591796875;0.103464211062779309902026625422877259552478790283203125;-0.70437804670905113102463701579836197197437286376953125;-0.0895531557611066453272741227920050732791423797607421875;0.9385866729123553131586277231690473854541778564453125;1.0586084917643123759489753865636885166168212890625;-0.20805475808848739038836583858937956392765045166015625;-0.0001208088106012937426418651920556612822110764682292938232421875;-0.11382711872823221554984485237582703121006488800048828125;0.046931263252700507193626577873146743513643741607666015625]
      mask Display: e = 0.06;c1 = [120 150 230]/255;c2 = ([120 150 230]+0)/383;c3 = ([120 150 230]+128)/383;patch([0 1 1 0],[0 0 1 1],c1);patch([0 1 1 1-e 1-e 0+e],[0 0 1 1-e 0+e 0+e],c2);patch([0 0 1 1-e 0+e 0+e],[0 1 1 1-e 1-e 0+e],c3);plot([0 1 1 0 0],[0 0 1 1 0]);disp('weights');
  Mux : Mux  Inputs=1
      mask Display: e = 0.06;c1 = [120 150 230]/255;c2 = ([120 150 230]+0)/383;c3 = ([120 150 230]+128)/383;patch([0 1 1 0],[0 0 1 1],c1);patch([0 1 1 1-e 1-e 0+e],[0 0 1 1-e 0+e 0+e],c2);patch([0 0 1 1-e 0+e 0+e],[0 1 1 1-e 1-e 0+e],c3);plot([0 1 1 0 0],[0 0 1 1 0]);disp('Mux');
  dotprod1 : neural/Weight Functions/dotprod
  "lz{2,1}" : Outport
      mask Display: e = 0.06;c1 = [120 230 180]/255;c2 = ([120 230 180]+0)/(256+128);c3 = ([120 230 180]+128)/(256+128);patch([0 1 1 0],[0 0 1 1],c1);patch([0 1 1 1-e 1-e 0+e],[0 0 1 1-e 0+e 0+e],c2);patch([0 0 1 1-e 0+e 0+e],[0 1 1 1-e 1-e 0+e],c3);plot([0 1 1 0 0],[0 0 1 1 0]);
  wires:
  "IW{2,1}(1,:)'"/1 -> dotprod1/1
  "ad{2,1}"/1 -> dotprod1/2
  dotprod1/1 -> Mux/1
  Mux/1 -> "lz{2,1}"/1

== system mrefrobotarm_modified_previous_y_previous_u_previous_ref_Thao/trimmed_2_report/Layer 1/Delays 1 ==
  "p{1}" : Inport  PortDimensions=10
      mask Display: e = 0.06;c1 = [120 230 180]/255;c2 = ([120 230 180]+0)/(256+128);c3 = ([120 230 180]+128)/(256+128);patch([0 1 1 0],[0 0 1 1],c1);patch([0 1 1 1-e 1-e 0+e],[0 0 1 1-e 0+e 0+e],c2);patch([0 0 1 1-e 0+e 0+e],[0 1 1 1-e 1-e 0+e],c3);plot([0 1 1 0 0],[0 0 1 1 0]);
  mux : Mux  Inputs=1
      mask Display: e = 0.06;c1 = [120 150 230]/255;c2 = ([120 150 230]+0)/383;c3 = ([120 150 230]+128)/383;patch([0 1 1 0],[0 0 1 1],c1);patch([0 1 1 1-e 1-e 0+e],[0 0 1 1-e 0+e 0+e],c2);patch([0 0 1 1-e 0+e 0+e],[0 1 1 1-e 1-e 0+e],c3);plot([0 1 1 0 0],[0 0 1 1 0]);disp('Mux')
  "pd{1,1}" : Outport
      mask Display: e = 0.06;c1 = [120 230 180]/255;c2 = ([120 230 180]+0)/(256+128);c3 = ([120 230 180]+128)/(256+128);patch([0 1 1 0],[0 0 1 1],c1);patch([0 1 1 1-e 1-e 0+e],[0 0 1 1-e 0+e 0+e],c2);patch([0 0 1 1-e 0+e 0+e],[0 1 1 1-e 1-e 0+e],c3);plot([0 1 1 0 0],[0 0 1 1 0]);
  wires:
  "p{1}"/1 -> mux/1
  mux/1 -> "pd{1,1}"/1
